simulink model "Model_Development"  (R2019a)
settings: Solver=FixedStepAuto  StartTime=0.0  StopTime=Inf  FixedStep=0.1  RelTol=1e-3
PostLoadFcn:
  | if any(exist('dsrtsu_mdlpostloadfcn', 'file') ~= 0), dsrtsu_mdlpostloadfcn('Execute', bdroot); end
InitFcn:
  | , if any(exist('rtifpga_mdlclblib', 'file') ~= 0), rtifpga_mdlclblib('Init', bdroot); end,
  | , if any(exist('dsmpb_private', 'file') ~= 0), dsmpb_private('dsmpb_mdlclblib', 'Init', bdroot); end,
libraries: dsmpblib x2
PreSaveFcn:
  | , if any(exist('dsmpb_private', 'file') ~= 0), dsmpb_private('dsmpb_mdlclblib', 'PreSave', bdroot); end,
CloseFcn:
  | , if any(exist('dsmpb_private', 'file') ~= 0), dsmpb_private('dsmpb_mdlclblib', 'Close', bdroot); end,
settings Model: DSMPB_ID_DATA={'28',struct('BlockId','9f1fea50-99ed-4d45-8ad3-952fb9fbb3f7','SignalIds',{{'3f5e9160-ecb2-4fe5-bf14-617dbef05cb2'}}),'31',struct('BlockId','10894696-7aac-4333-a05e-37f13e0eedfc','SignalIds',{{'d61dd94f-0b03-43b6-9401-8b62f8eb8c9e','703cc474-4f8c-426e-980c-7f3b47c6f237','283ba769-de60-4e66-8dae-9c9288764590','6a7dd420-ff6f-4b9d-b626-112f75dcf41e','74e8e34e-38ec-4726-b97a-e21645c081c3'}})}  RTICANMMDATA=struct('GeneralSetupData',struct('modelroot','C:\Users\RCP-Lab\Documents\00_Projekte\00_MODEL\Development_Ajay','generalsettings',struct('filesettings',struct('destfolder',struct('Name','RTICANMM_FILES','Check',1),'buildfolder',struct('Name','.','Check',1),'AbsDestfolder',struct('Name','C:\Users\RCP-Lab\Documents\00_Projekte\00_MODEL\Development_Ajay\RTICANMM_FILES'),'AbsBuildfolder',struct('Name','C:\Users\RCP-Lab\Documents\00_Projekte\00_MODEL\Development_Ajay'))),'options',struct('addpaths',1,'rmpaths',1,'addtrcexclusion',true,'cannavigator',struct('checkmonitoring',0),'show_usrtrc',0,'use_usrtrc',0),'advanced',struct('options',ones(1,100)),'MPSetup',{{}},'RTI',struct('Type','DSRT','Ver','4.3','Date','02-May-2020'),'modelname','Model_Development','block','Model_Development'))  DSRTSU_INTERNAL_RTIFPGA=160  Creator=RCP-Lab  LastModifiedBy=RCP-Lab
settings OptimizationCC: BlockReduction=off  ConditionallyExecuteInputs=off  OptimizeBlockIOStorage=off  BufferReuse=off  GlobalBufferReuse=off  ExpressionFolding=off  LocalBlockOutputs=off  OptimizeDataStoreBuffers=off  BusAssignmentInplaceUpdate=off
settings DebuggingCC: TasksWithSamePriorityMsg=none
settings HardwareCC: ProdBitPerPointer=32  ProdBitPerSizeT=32  ProdBitPerPtrDiffT=32  ProdLargestAtomicInteger=Integer  ProdWordSize=32  ProdLongLongMode=on  ProdHWDeviceType=Custom Processor->Custom
settings ModelReferenceCC: EnableParallelModelReferenceBuilds=on
settings SFSimCC: MATLABDynamicMemAlloc=off
settings RTWCC: SystemTargetFile=dsrt.tlc  GenCodeOnly=on  MakeCommand=make_dsrt  TemplateMakefile=dsrt_default_tmf  Description=dSPACE Run-Time Target (for VEOS on Windows and ConfigurationDesk)  RTWVerbose=off
settings STFCustomTargetCC: TargetLangStandard=C99 (ISO)  ParMdlRefBuildCompliant=on  GRTInterface=off  SystemTargetFile=dsrt.tlc
settings GRTTargetCC: CompOptLevelCompliant=off  ConcurrentExecutionCompliant=off  CombineOutputUpdateFcns=off  MatFileLogging=off  CPPClassGenCompliant=off  UseToolchainInfoCompliant=off

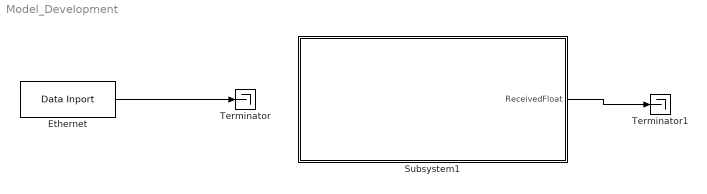
== system Model_Development ==
  Ethernet : dsmpblib/Data Inport  Priority=10000
      settings: SourceProductName=dSPACE Model Interface Blockset
  Subsystem1 : Subsystem
  Terminator : Terminator
  Terminator1 : Terminator
  wires:
  Ethernet/1 -> Terminator/1
  Subsystem1/1(ReceivedFloat) -> Terminator1/1

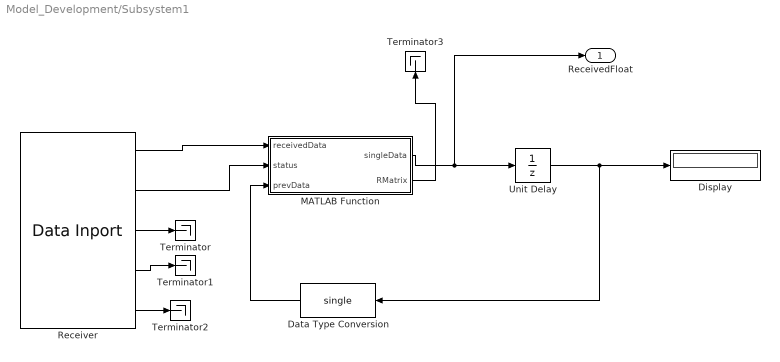
== system Model_Development/Subsystem1 ==
  Data Type Conversion : DataTypeConversion  OutMin=[1]  OutMax=[1]  OutDataTypeStr=single
  Display : Display
      settings: Format=decimal (Stored Integer)
  MATLAB Function : MATLAB Function  TreatAsAtomicUnit=on
  Receiver : dsmpblib/Data Inport  Priority=10000
      settings: SourceProductName=dSPACE Model Interface Blockset
  Terminator{,1..3} (4 alike) : Terminator
  Unit Delay : UnitDelay  InitialCondition=single(0)  SampleTime=-1  HasFrameUpgradeWarning=on
  ReceivedFloat : Outport
  wires:
  Data Type Conversion/1 -> MATLAB Function/3(prevData)
  Unit Delay/1 -> Data Type Conversion/1, Display/1
  Receiver/2 -> MATLAB Function/2(status)
  MATLAB Function/1(singleData) -> Unit Delay/1, ReceivedFloat/1
  Receiver/1 -> MATLAB Function/1(receivedData)
  Receiver/3 -> Terminator/1
  Receiver/4 -> Terminator1/1
  Receiver/5 -> Terminator2/1
  MATLAB Function/2(RMatrix) -> Terminator3/1

== matlab function Model_Development/Subsystem1/MATLAB Function ==
  data: receivedData input; singleData output; status input; prevData input; RMatrix output size=1000
function [singleData, RMatrix] = convertToSingleWithHold(receivedData,   status, prevData)
    % Convert received data to single precision and retain previous value if no new data
    %
    % Inputs:
    %   receivedData - Input data (e.g., double, uint8, etc.)
    %   status       - Status flag (1 = process data, 0 = hold previous value)
    %   prevData     - Previous output value (fed back into the function)
    %
    % Outputs:
    %   singleData   - Data converted to single precision or retained previous value

    persistent rows cols currentRow currentCol matrix;
    %coder.varsize('RMatrix',[1000,1000]);
    RMatrix = zeros(1, 1);
    %receivedData = all(receivedData);
    %receivedData = typecast(receivedData, 'single');
    % Check if prevData is empty (first iteration)
    if isempty(prevData)
        % Initialize singleData with a default value
        singleData = single(-1); % Default initialization
        return;
    end

     %Initialize persistent variables
    if isempty(rows) || (all(receivedData) == -1  && status == 1)
        rows = single(-1);          % Initialize rows as -1
        cols = single(-1);          % Initialize cols as -1
        currentRow = 1;     % Start filling from the first row
        currentCol = 1;     % Start filling from the first column
        matrix = zeros(1, 1);        % Initialize matrix as empty
        singleData = single(0);
        return
    end

    

    if status == 1
        if rows == -1
            % If rows are not set, set rows from received data
            rows = typecast(receivedData, 'single');
            %rows = typecast(all(receivedData), 'single');  % Decode float32 value for rows
            singleData = typecast(receivedData, 'single');
            return;
        elseif cols == -1
            % If cols are not set, set cols from received data
            cols = typecast(receivedData, 'single');
            %cols = typecast(all(receivedData), 'single');  % Decode float32 value for cols
            assert(rows <= 1000 && cols <= 1000,'Size exceeds');
            matrix = zeros(rows, cols);              % Preallocate matrix after dimensions are known
            singleData = typecast(receivedData, 'single');
            return;
        else
            % Process incoming data and fill the matrix row by row, column by column
            singleData = typecast(receivedData, 'single');
            %singleData = typecast(all(receivedData), 'single');  % Decode float32 value
            
            if currentRow <= rows && currentCol <= cols
                matrix(currentRow, currentCol) = singleData;  % Fill the current cell in the matrix
                
                % Move to the next column or row when a row is complete
                currentCol = currentCol + 1;
                if currentCol > cols
                    currentCol = 1;          % Reset column index to 1
                    currentRow = currentRow + 1;  % Move to the next row
                    
                    if currentRow > rows
                        disp("Matrix reconstruction complete!");
                        disp(matrix);       % Display the reconstructed matrix in Command Window
                        %RMatrix = reshape([], [rows,cols]);
                        RMatrix = matrix;

                        % Reset persistent variables for the next cycle
                        rows = single(-1);
                        cols = single(-1);
                        currentRow = 1;
                        currentCol = 1;
                        singleData = single(0);  % Reset output to default value
                        return;
                    end
                end
            end
        end
    else
        % If no new data, retain the previous value
        singleData = single(prevData);
    end
end
